simulink model "motor"  (R2024b)
settings: Solver=VariableStepAuto  StartTime=0.0  StopTime=3  RelTol=1e-3
settings Model: Creator=crunc  LastModifiedBy=crunc

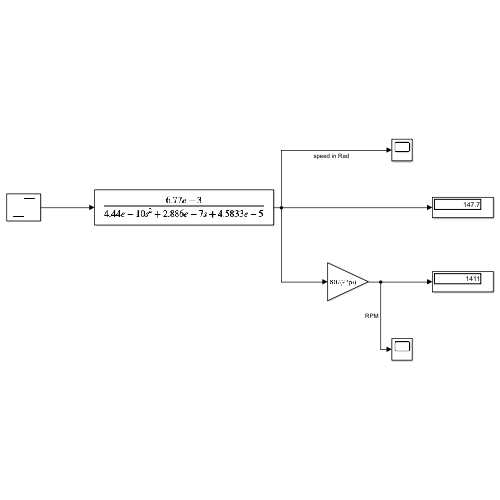
[thumbnail: Simulink's stored preview of the top-level diagram]
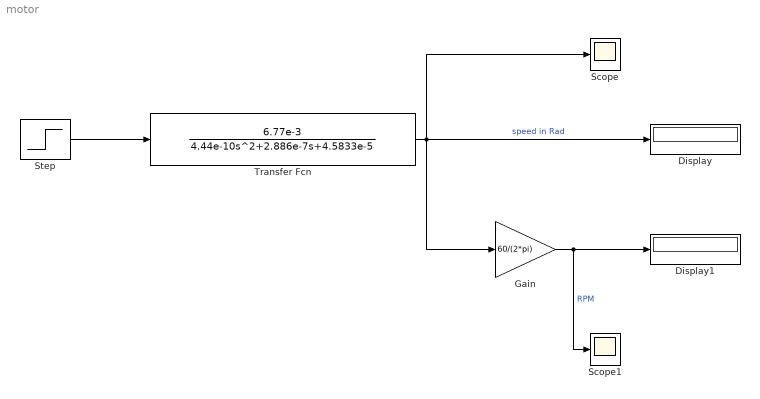
== system motor ==
  Display : Display
  Display1 : Display
  Gain : Gain  Gain=60/(2*pi)
  Scope : Scope
  Scope1 : Scope
  Step : Step  SampleTime=0
  Transfer Fcn : TransferFcn  Numerator=[6.77e-3]  Denominator=[4.44e-10 2.886e-7 4.5833e-5]
  wires:
  Step/1 -> Transfer Fcn/1
  Transfer Fcn/1 -> Display/1, Scope/1, Gain/1  "speed in Rad"
  Gain/1 -> Scope1/1, Display1/1  "RPM"
